simulink model "ROS"  (R2020b)
settings: Solver=FixedStepDiscrete  StartTime=start  StopTime=stop  FixedStep=T  MaxStep=0.01  RelTol=1e-3  EnableMultiTasking=on
model workspace (MAT data in the model file):
  SL_ROS_VariableLengthArrays_MaxSizes.CommonInfo.ArrayTruncateAction = 'EmitWarning'
  SL_ROS_VariableLengthArrays_MaxSizes.MsgTypeMap = containers.Map
  SL_ROS_VariableLengthArrays_MaxSizes.MsgTypeMap.serialization.keys = {'mav_msgs/Actuators'}
  SL_ROS_VariableLengthArrays_MaxSizes.MsgTypeMap.serialization.values{1}(1).PropertyName = 'Angles'
  SL_ROS_VariableLengthArrays_MaxSizes.MsgTypeMap.serialization.values{1}(1).DataType = 'double'
  SL_ROS_VariableLengthArrays_MaxSizes.MsgTypeMap.serialization.values{1}(1).MaxLength = 128
  SL_ROS_VariableLengthArrays_MaxSizes.MsgTypeMap.serialization.values{1}(2).PropertyName = 'AngularVelocities'
  SL_ROS_VariableLengthArrays_MaxSizes.MsgTypeMap.serialization.values{1}(2).DataType = 'double'
  SL_ROS_VariableLengthArrays_MaxSizes.MsgTypeMap.serialization.values{1}(2).MaxLength = 6
  SL_ROS_VariableLengthArrays_MaxSizes.MsgTypeMap.serialization.values{1}(3).PropertyName = 'Normalized'
  SL_ROS_VariableLengthArrays_MaxSizes.MsgTypeMap.serialization.values{1}(3).DataType = 'double'
  SL_ROS_VariableLengthArrays_MaxSizes.MsgTypeMap.serialization.values{1}(3).MaxLength = 128
  SL_ROS_VariableLengthArrays_MaxSizes.MsgTypeMap.serialization.uniformity = 0
  SL_ROS_VariableLengthArrays_MaxSizes.MsgTypeMap.serialization.keyType = 'char'
  SL_ROS_VariableLengthArrays_MaxSizes.MsgTypeMap.serialization.valueType = 'any'
values from neighbouring files (symbols this model uses):
  deltaOmegaNegBound = -1718    [ROS_Controller_Example.m]
  deltaOmegaPosBound = 1289    [ROS_Controller_Example.m]
  intAttPhi = intAttPhi_SIMULINK.signals.values(end)    [ROS_Controller_Example.m]
  intAttTheta = intAttTheta_SIMULINK.signals.values(end)    [ROS_Controller_Example.m]
  intPosXX = intPosXX_SIMULINK.signals.values(end)    [ROS_Controller_Example.m]
  intPosYY = intPosYY_SIMULINK.signals.values(end)    [ROS_Controller_Example.m]
  intRateRate = intRateRate_SIMULINK.signals.values(end)    [ROS_Controller_Example.m]
  intZZ = intZZ_SIMULINK.signals.values(end)    [ROS_Controller_Example.m]
  Kd_altitude = 373    [ROS_Controller_Example.m]
  Ki_altitude = 3.15    [ROS_Controller_Example.m]
  Ki_deltaPsi = 95.6839    [ROS_Controller_Example.m]
  Ki_pc = 0.0349    [ROS_Controller_Example.m]
  Ki_PhiC = -5.72958    [ROS_Controller_Example.m]
  Ki_qc = 0.0349    [ROS_Controller_Example.m]
  Ki_ThetaC = 5.72958    [ROS_Controller_Example.m]
  Kp_altitude = 70    [ROS_Controller_Example.m]
  Kp_deltaPhi = 1000    [ROS_Controller_Example.m]
  Kp_deltaPsi = 1000    [ROS_Controller_Example.m]
  Kp_deltaTheta = 1000    [ROS_Controller_Example.m]
  Kp_pc = 0.0611    [ROS_Controller_Example.m]
  Kp_PhiC = -3.594    [ROS_Controller_Example.m]
  Kp_qc = 0.0611    [ROS_Controller_Example.m]
  Kp_ThetaC = 3.594    [ROS_Controller_Example.m]
  Kp_YawPositionController = 0.0914    [ROS_Controller_Example.m]
  maxRotorsVelocity = 2618    [ROS_Controller_Example.m]
  motorAngularCoefficient = 0.2685    [ROS_Controller_Example.m]
  motorsIntercepts = 426.24    [ROS_Controller_Example.m]
  Omega_e = 6874    [ROS_Controller_Example.m]
  p_GAZEBO = msgS.Twist.Twist.Angular.X    [ROS_Controller_Example.m]
  phiCBound = pi/6    (= 0.523598775598)    [ROS_Controller_Example.m]
  pitch_MATLAB = EulerAngles(1,2)    [ROS_Controller_Example.m]
  psi_ref = 0    [ROS_Controller_Example.m]
  q_GAZEBO = msgS.Twist.Twist.Angular.Y    [ROS_Controller_Example.m]
  r_GAZEBO = msgS.Twist.Twist.Angular.Z    [ROS_Controller_Example.m]
  roll_MATLAB = EulerAngles(1,3)    [ROS_Controller_Example.m]
  T = 0.01    [ROS_Controller_Example.m]
  thetaCBound = pi/6    (= 0.523598775598)    [ROS_Controller_Example.m]
  u_GAZEBO = msgS.Twist.Twist.Linear.X    [ROS_Controller_Example.m]
  v_GAZEBO = msgS.Twist.Twist.Linear.Y    [ROS_Controller_Example.m]
  w_GAZEBO = msgS.Twist.Twist.Linear.Z    [ROS_Controller_Example.m]
  x_GAZEBO = msgS.Pose.Pose.Position.X    [ROS_Controller_Example.m]
  x_ref = 0    [ROS_Controller_Example.m]
  y_GAZEBO = msgS.Pose.Pose.Position.Y    [ROS_Controller_Example.m]
  y_ref = 0    [ROS_Controller_Example.m]
  yaw_MATLAB = EulerAngles(1,1)    [ROS_Controller_Example.m]
  yawRateBound = 3.4907    [ROS_Controller_Example.m]
  z_GAZEBO = msgS.Pose.Pose.Position.Z    [ROS_Controller_Example.m]
  z_ref = 1    [ROS_Controller_Example.m]
undefined symbols (not defined in the file or in its folder): DiscIntNeverNeededParam
settings Model: Creator=giuse  LastModifiedBy=FranciscoJose
settings DataIOCC: LimitDataPoints=on  SaveFormat=Array  ReturnWorkspaceOutputs=off
settings OptimizationCC: MaxStackSize=64
settings DebuggingCC: ParameterTunabilityLossMsg=error  ArithmeticOperatorsInVariantConditions=warning
settings HardwareCC: ProdBitPerPointer=32  ProdBitPerSizeT=32  ProdBitPerPtrDiffT=32  ProdLargestAtomicFloat=None  ProdIntDivRoundTo=Undefined  ProdEndianess=Unspecified  ProdWordSize=32  ProdHWDeviceType=Generic->Unspecified (assume 32-bit Generic)  UseEmbeddedCoderFeatures=off
settings ModelReferenceCC: PropagateSignalLabelsOutOfModel=off
settings SFSimCC: SimUseLocalCustomCode=off  CustomCodeUndefinedFunction=UseInterfaceOnly  SimTargetLang=C++
settings RTWCC: Description=Embedded Coder  SystemTargetFile=ert.tlc  HardwareBoard=Robot Operating System (ROS)  TLCOptions="-aInlineSetEventsForThisBaseRateFcn=TLC_FALSE -aSuppressMultiTaskScheduler=TLC_FALSE  -aRateBasedStepFcn=0"  TemplateMakefile=ert_default_tmf  GenerateReport=on  RTWUseLocalCustomCode=off  Toolchain=Catkin  LaunchReport=on  TargetLang=C++
settings CodeAppCC: ForceParamTrailComments=on  OperatorAnnotations=on  StateflowObjectComments=on  MATLABSourceComments=on
settings ERTTargetCC: MultiwordLength=2048  ERTCustomFileBanners=off  SupportContinuousTime=on  SupportNonInlinedSFcns=on  RemoveResetFunc=off  ModelStepFunctionPrototypeControlCompliant=off

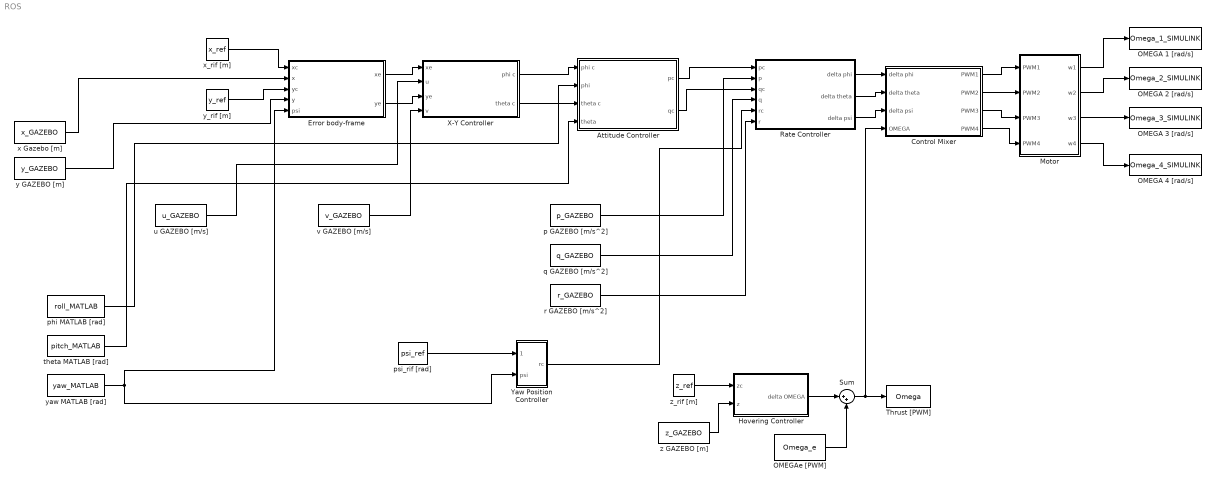
== system ROS ==
  Attitude Controller : Subsystem
  Control Mixer : Subsystem
  Error body-frame : Subsystem
  Hovering Controller : Subsystem
  Motor : Subsystem
  OMEGA 1 [rad/s] : ToWorkspace  VariableName=Omega_1_SIMULINK  SaveFormat=Structure With Time  SampleTime=-1
  OMEGA 2 [rad/s] : ToWorkspace  VariableName=Omega_2_SIMULINK  SaveFormat=Structure With Time  SampleTime=-1
  OMEGA 3 [rad/s] : ToWorkspace  VariableName=Omega_3_SIMULINK  SaveFormat=Structure With Time  SampleTime=-1
  OMEGA 4 [rad/s] : ToWorkspace  VariableName=Omega_4_SIMULINK  SaveFormat=Structure With Time  SampleTime=-1
  OMEGAe [PWM] : Constant  Value=Omega_e
  Rate Controller : Subsystem
  Sum : Sum  Inputs=|++
  Thrust [PWM] : ToWorkspace  VariableName=Omega  SaveFormat=Structure With Time  SampleTime=-1
  X-Y Controller : Subsystem
  Yaw Position Controller : Subsystem
  p GAZEBO [m/s^2] : Constant  Value=p_GAZEBO
  phi MATLAB [rad] : Constant  Value=roll_MATLAB
  psi_rif [rad] : Constant  Value=psi_ref
  q GAZEBO [m/s^2] : Constant  Value=q_GAZEBO
  r GAZEBO [m/s^2] : Constant  Value=r_GAZEBO
  theta MATLAB [rad] : Constant  Value=pitch_MATLAB
  u GAZEBO [m/s] : Constant  Value=u_GAZEBO
  v GAZEBO [m/s] : Constant  Value=v_GAZEBO
  x Gazebo [m] : Constant  Value=x_GAZEBO
  x_rif [m] : Constant  Value=x_ref
  y GAZEBO [m] : Constant  Value=y_GAZEBO
  y_rif [m] : Constant  Value=y_ref
  yaw MATLAB [rad] : Constant  Value=yaw_MATLAB
  z GAZEBO [m] : Constant  Value=z_GAZEBO
  z_rif [m] : Constant  Value=z_ref
  wires:
  Attitude Controller/2(qc) -> Rate Controller/3(qc)
  Control Mixer/1(PWM1) -> Motor/1(PWM1)
  Attitude Controller/1(pc) -> Rate Controller/1(pc)
  Control Mixer/2(PWM2) -> Motor/2(PWM2)
  Control Mixer/3(PWM3) -> Motor/3(PWM3)
  Control Mixer/4(PWM4) -> Motor/4(PWM4)
  Rate Controller/1(delta phi) -> Control Mixer/1(delta phi)
  Rate Controller/2(delta theta) -> Control Mixer/2(delta theta)
  Yaw Position Controller/1(rc) -> Rate Controller/5(rc)
  yaw MATLAB [rad]/1 -> Yaw Position Controller/2(psi), Error body-frame/5(psi)
  psi_rif [rad]/1 -> Yaw Position Controller/1(psi c)
  q GAZEBO [m/s^2]/1 -> Rate Controller/4(q)
  phi MATLAB [rad]/1 -> Attitude Controller/2(phi)
  z_rif [m]/1 -> Hovering Controller/1(zc)
  y_rif [m]/1 -> Error body-frame/3(yc)
  X-Y Controller/2(theta c) -> Attitude Controller/3(theta c)
  r GAZEBO [m/s^2]/1 -> Rate Controller/6(r)
  OMEGAe [PWM]/1 -> Sum/2
  X-Y Controller/1(phi c) -> Attitude Controller/1(phi c)
  Error body-frame/1(xe) -> X-Y Controller/1(xe)
  Hovering Controller/1(delta OMEGA) -> Sum/1
  Error body-frame/2(ye) -> X-Y Controller/3(ye)
  p GAZEBO [m/s^2]/1 -> Rate Controller/2(p)
  theta MATLAB [rad]/1 -> Attitude Controller/4(theta)
  x_rif [m]/1 -> Error body-frame/1(xc)
  Rate Controller/3(delta psi) -> Control Mixer/3(delta psi)
  Sum/1 -> Control Mixer/4(OMEGA), Thrust [PWM]/1
  x Gazebo [m]/1 -> Error body-frame/2(x)
  y GAZEBO [m]/1 -> Error body-frame/4(y)
  z GAZEBO [m]/1 -> Hovering Controller/2(z)
  u GAZEBO [m/s]/1 -> X-Y Controller/2(u)
  v GAZEBO [m/s]/1 -> X-Y Controller/4(v)
  Motor/3(w3) -> OMEGA 3 [rad/s]/1
  Motor/4(w4) -> OMEGA 4 [rad/s]/1
  Motor/2(w2) -> OMEGA 2 [rad/s]/1
  Motor/1(w1) -> OMEGA 1 [rad/s]/1

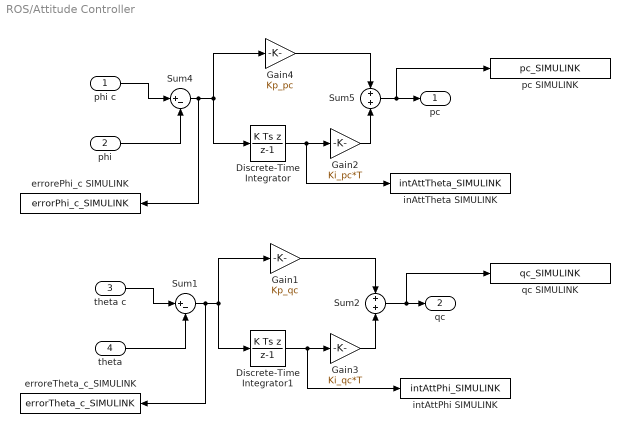
== system ROS/Attitude Controller ==
  phi c : Inport
  phi : Inport  Port=2
  theta c : Inport  Port=3
  theta : Inport  Port=4
  Discrete-Time Integrator : DiscreteIntegrator  IntegratorMethod=Integration: Backward Euler  gainval=1  InitialCondition=intAttPhi  SampleTime=-1  ICPrevOutput=DiscIntNeverNeededParam  ICPrevScaledInput=DiscIntNeverNeededParam
  Discrete-Time Integrator1 : DiscreteIntegrator  IntegratorMethod=Integration: Backward Euler  gainval=1  InitialCondition=intAttTheta  SampleTime=-1  ICPrevOutput=DiscIntNeverNeededParam  ICPrevScaledInput=DiscIntNeverNeededParam
  Gain1 : Gain  Gain=Kp_qc
  Gain2 : Gain  Gain=Ki_pc*T
  Gain3 : Gain  Gain=Ki_qc*T
  Gain4 : Gain  Gain=Kp_pc
  Sum1 : Sum  Inputs=|+-
  Sum2 : Sum
  Sum4 : Sum  Inputs=|+-
  Sum5 : Sum
  errorePhi_c SIMULINK : ToWorkspace  VariableName=errorPhi_c_SIMULINK  SaveFormat=Structure With Time  SampleTime=-1
  erroreTheta_c_SIMULINK : ToWorkspace  VariableName=errorTheta_c_SIMULINK  SaveFormat=Structure With Time  SampleTime=-1
  inAttTheta SIMULINK : ToWorkspace  VariableName=intAttTheta_SIMULINK  SaveFormat=Structure With Time  SampleTime=-1
  intAttPhi SIMULINK : ToWorkspace  VariableName=intAttPhi_SIMULINK  SaveFormat=Structure With Time  SampleTime=-1
  pc SIMULINK : ToWorkspace  VariableName=pc_SIMULINK  SaveFormat=Structure With Time  SampleTime=-1
  qc SIMULINK : ToWorkspace  VariableName=qc_SIMULINK  SaveFormat=Structure With Time  SampleTime=-1
  pc : Outport  VectorParamsAs1DForOutWhenUnconnected=off
  qc : Outport  Port=2  VectorParamsAs1DForOutWhenUnconnected=off
  wires:
  Gain4/1 -> Sum5/1
  Sum4/1 -> errorePhi_c SIMULINK/1, Discrete-Time Integrator/1, Gain4/1
  phi/1 -> Sum4/2
  Discrete-Time Integrator/1 -> inAttTheta SIMULINK/1, Gain2/1
  phi c/1 -> Sum4/1
  Sum5/1 -> pc SIMULINK/1, pc/1
  Gain1/1 -> Sum2/1
  Sum1/1 -> erroreTheta_c_SIMULINK/1, Discrete-Time Integrator1/1, Gain1/1
  theta/1 -> Sum1/2
  theta c/1 -> Sum1/1
  Sum2/1 -> qc SIMULINK/1, qc/1
  Gain2/1 -> Sum5/2
  Gain3/1 -> Sum2/2
  Discrete-Time Integrator1/1 -> intAttPhi SIMULINK/1, Gain3/1

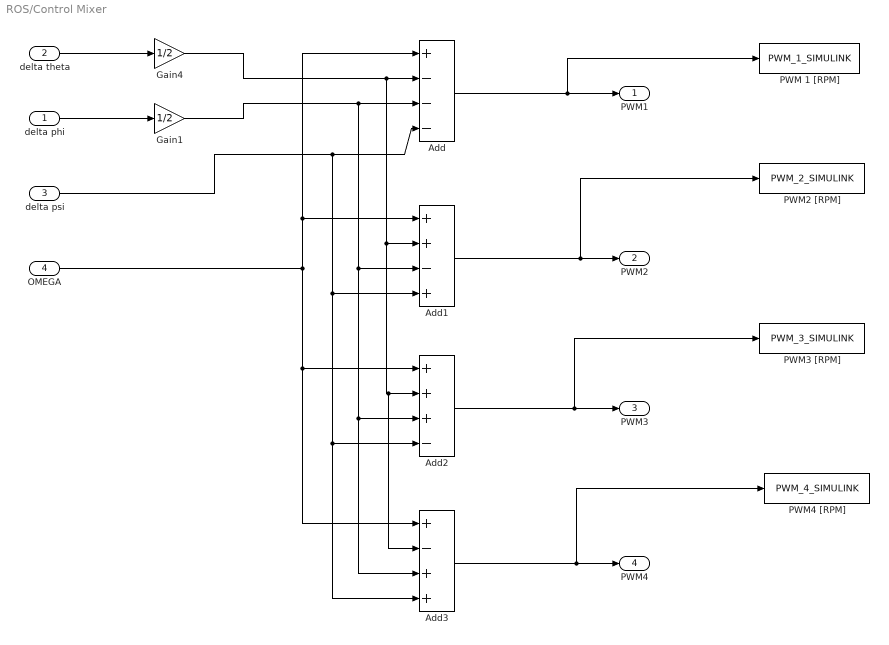
== system ROS/Control Mixer ==
  delta phi : Inport
  delta theta : Inport  Port=2
  delta psi : Inport  Port=3
  OMEGA : Inport  Port=4
  Add : Sum  Inputs=+---
  Add1 : Sum  Inputs=++-+
  Add2 : Sum  Inputs=+++-
  Add3 : Sum  Inputs=+-++
  Gain1 : Gain  Gain=1/2
  Gain4 : Gain  Gain=1/2
  PWM 1 [RPM] : ToWorkspace  VariableName=PWM_1_SIMULINK  SaveFormat=Structure With Time  SampleTime=-1
  PWM2 [RPM] : ToWorkspace  VariableName=PWM_2_SIMULINK  SaveFormat=Structure With Time  SampleTime=-1
  PWM3 [RPM] : ToWorkspace  VariableName=PWM_3_SIMULINK  SaveFormat=Structure With Time  SampleTime=-1
  PWM4 [RPM] : ToWorkspace  VariableName=PWM_4_SIMULINK  SaveFormat=Structure With Time  SampleTime=-1
  PWM1 : Outport  VectorParamsAs1DForOutWhenUnconnected=off
  PWM2 : Outport  Port=2  VectorParamsAs1DForOutWhenUnconnected=off
  PWM3 : Outport  Port=3  VectorParamsAs1DForOutWhenUnconnected=off
  PWM4 : Outport  Port=4  VectorParamsAs1DForOutWhenUnconnected=off
  wires:
  delta phi/1 -> Gain1/1
  OMEGA/1 -> Add1/1, Add/1, Add3/1, Add2/1
  Gain4/1 -> Add/2, Add1/2, Add3/2, Add2/2
  delta theta/1 -> Gain4/1
  delta psi/1 -> Add3/4, Add2/4, Add1/4, Add/4
  Gain1/1 -> Add/3, Add1/3, Add3/3, Add2/3
  Add/1 -> PWM 1 [RPM]/1, PWM1/1
  Add1/1 -> PWM2 [RPM]/1, PWM2/1
  Add2/1 -> PWM3 [RPM]/1, PWM3/1
  Add3/1 -> PWM4 [RPM]/1, PWM4/1

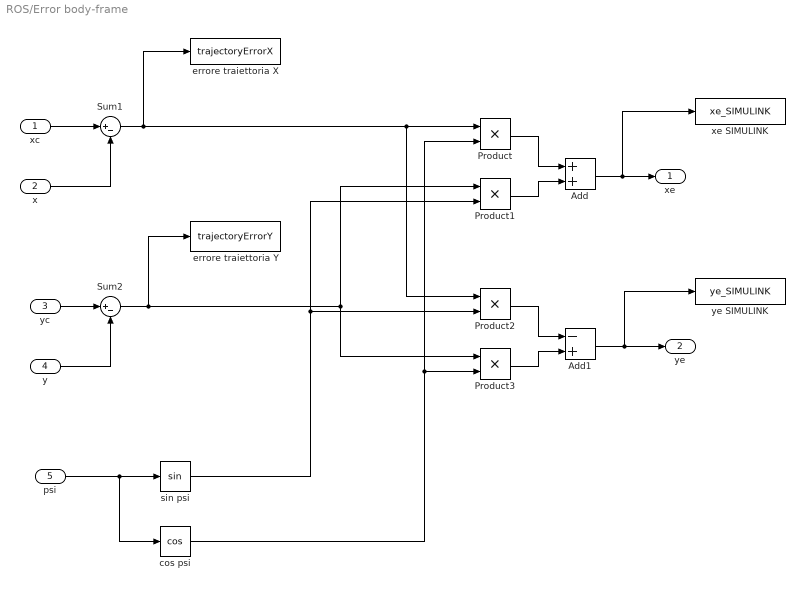
== system ROS/Error body-frame ==
  xc : Inport
  x : Inport  Port=2
  yc : Inport  Port=3
  y : Inport  Port=4
  psi : Inport  Port=5
  Add : Sum
  Add1 : Sum  Inputs=-+
  Product{,1..3} (4 alike) : Product
  Sum1 : Sum  Inputs=|+-
  Sum2 : Sum  Inputs=|+-
  cos psi : Trigonometry  Operator=cos
  errore traiettoria X : ToWorkspace  VariableName=trajectoryErrorX  SaveFormat=Structure With Time  SampleTime=-1
  errore traiettoria Y : ToWorkspace  VariableName=trajectoryErrorY  SaveFormat=Structure With Time  SampleTime=-1
  sin psi : Trigonometry
  xe SIMULINK : ToWorkspace  VariableName=xe_SIMULINK  SaveFormat=Structure With Time  SampleTime=-1
  ye SIMULINK : ToWorkspace  VariableName=ye_SIMULINK  SaveFormat=Structure With Time  SampleTime=-1
  xe : Outport  VectorParamsAs1DForOutWhenUnconnected=off
  ye : Outport  Port=2  VectorParamsAs1DForOutWhenUnconnected=off
  wires:
  x/1 -> Sum1/2
  xc/1 -> Sum1/1
  y/1 -> Sum2/2
  yc/1 -> Sum2/1
  psi/1 -> sin psi/1, cos psi/1
  Product1/1 -> Add/2
  Product/1 -> Add/1
  Product3/1 -> Add1/2
  Product2/1 -> Add1/1
  Sum1/1 -> errore traiettoria X/1, Product2/1, Product/1
  Sum2/1 -> Product3/1, Product1/1, errore traiettoria Y/1
  Add1/1 -> ye SIMULINK/1, ye/1
  Add/1 -> xe SIMULINK/1, xe/1
  cos psi/1 -> Product3/2, Product/2
  sin psi/1 -> Product2/2, Product1/2

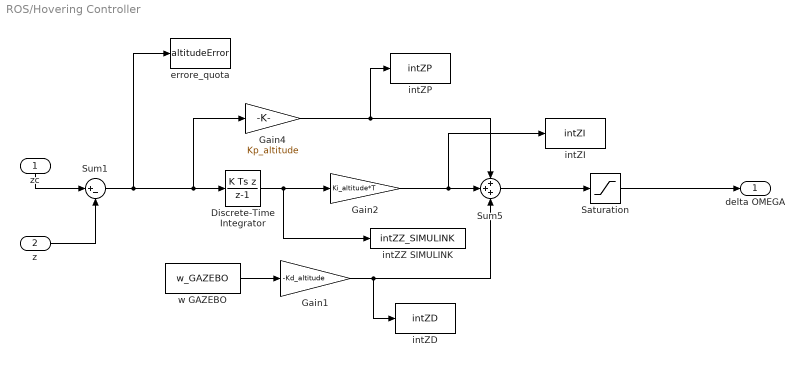
== system ROS/Hovering Controller ==
  zc : Inport
  z : Inport  Port=2
  Discrete-Time Integrator : DiscreteIntegrator  IntegratorMethod=Integration: Backward Euler  gainval=1  InitialCondition=intZZ  SampleTime=-1  ICPrevOutput=DiscIntNeverNeededParam  ICPrevScaledInput=DiscIntNeverNeededParam
  Gain1 : Gain  Gain=-Kd_altitude
  Gain2 : Gain  Gain=Ki_altitude*T
  Gain4 : Gain  Gain=Kp_altitude
  Saturation : Saturate  UpperLimit=deltaOmegaPosBound  LowerLimit=deltaOmegaNegBound
  Sum1 : Sum  Inputs=|+-
  Sum5 : Sum  Inputs=+++
  errore_quota : ToWorkspace  VariableName=altitudeError  SaveFormat=Structure With Time  SampleTime=-1
  intZD : ToWorkspace  VariableName=intZD  SaveFormat=Structure With Time  SampleTime=-1
  intZI : ToWorkspace  VariableName=intZI  SaveFormat=Structure With Time  SampleTime=-1
  intZP : ToWorkspace  VariableName=intZP  SaveFormat=Structure With Time  SampleTime=-1
  intZZ SIMULINK : ToWorkspace  VariableName=intZZ_SIMULINK  SaveFormat=Structure With Time  SampleTime=-1
  w GAZEBO : Constant  Value=w_GAZEBO
  delta OMEGA : Outport  VectorParamsAs1DForOutWhenUnconnected=off
  wires:
  Sum1/1 -> errore_quota/1, Discrete-Time Integrator/1, Gain4/1
  Gain4/1 -> intZP/1, Sum5/1
  z/1 -> Sum1/2
  zc/1 -> Sum1/1
  Gain1/1 -> intZD/1, Sum5/3
  Sum5/1 -> Saturation/1
  w GAZEBO/1 -> Gain1/1
  Saturation/1 -> delta OMEGA/1
  Discrete-Time Integrator/1 -> intZZ SIMULINK/1, Gain2/1
  Gain2/1 -> intZI/1, Sum5/2

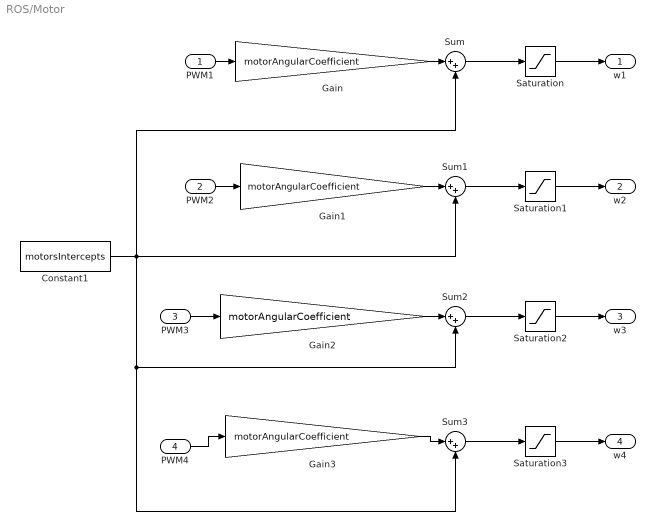
== system ROS/Motor ==
  PWM1 : Inport
  PWM2 : Inport  Port=2
  PWM3 : Inport  Port=3
  PWM4 : Inport  Port=4
  Constant1 : Constant  Value=motorsIntercepts
  Gain{,1..3} (4 alike) : Gain  Gain=motorAngularCoefficient
  Saturation{,1..3} (4 alike) : Saturate  UpperLimit=maxRotorsVelocity  LowerLimit=0
  Sum{,1..3} (4 alike) : Sum  Inputs=|++
  w1 : Outport  VectorParamsAs1DForOutWhenUnconnected=off
  w2 : Outport  Port=2  VectorParamsAs1DForOutWhenUnconnected=off
  w3 : Outport  Port=3  VectorParamsAs1DForOutWhenUnconnected=off
  w4 : Outport  Port=4  VectorParamsAs1DForOutWhenUnconnected=off
  wires:
  Gain/1 -> Sum/1
  PWM1/1 -> Gain/1
  Gain1/1 -> Sum1/1
  PWM2/1 -> Gain1/1
  Gain2/1 -> Sum2/1
  PWM3/1 -> Gain2/1
  Gain3/1 -> Sum3/1
  PWM4/1 -> Gain3/1
  Constant1/1 -> Sum1/2, Sum2/2, Sum3/2, Sum/2
  Sum/1 -> Saturation/1
  Sum1/1 -> Saturation1/1
  Sum2/1 -> Saturation2/1
  Sum3/1 -> Saturation3/1
  Saturation/1 -> w1/1
  Saturation1/1 -> w2/1
  Saturation2/1 -> w3/1
  Saturation3/1 -> w4/1

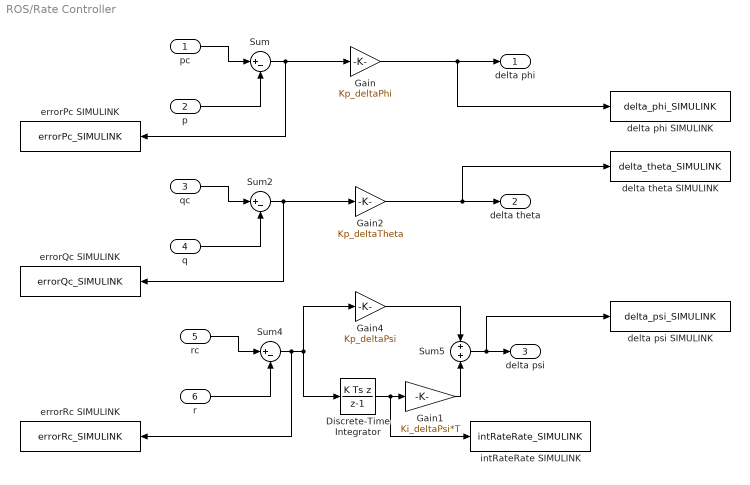
== system ROS/Rate Controller ==
  pc : Inport
  p : Inport  Port=2
  qc : Inport  Port=3
  q : Inport  Port=4
  rc : Inport  Port=5
  r : Inport  Port=6
  Discrete-Time Integrator : DiscreteIntegrator  IntegratorMethod=Integration: Backward Euler  gainval=1  InitialCondition=intRateRate  SampleTime=-1  ICPrevOutput=DiscIntNeverNeededParam  ICPrevScaledInput=DiscIntNeverNeededParam
  Gain : Gain  Gain=Kp_deltaPhi
  Gain1 : Gain  Gain=Ki_deltaPsi*T
  Gain2 : Gain  Gain=Kp_deltaTheta
  Gain4 : Gain  Gain=Kp_deltaPsi
  Sum : Sum  Inputs=|+-
  Sum2 : Sum  Inputs=|+-
  Sum4 : Sum  Inputs=|+-
  Sum5 : Sum
  delta phi SIMULINK : ToWorkspace  VariableName=delta_phi_SIMULINK  SaveFormat=Structure With Time  SampleTime=-1
  delta psi SIMULINK : ToWorkspace  VariableName=delta_psi_SIMULINK  SaveFormat=Structure With Time  SampleTime=-1
  delta theta SIMULINK : ToWorkspace  VariableName=delta_theta_SIMULINK  SaveFormat=Structure With Time  SampleTime=-1
  errorPc SIMULINK : ToWorkspace  VariableName=errorPc_SIMULINK  SaveFormat=Structure With Time  SampleTime=-1
  errorQc SIMULINK : ToWorkspace  VariableName=errorQc_SIMULINK  SaveFormat=Structure With Time  SampleTime=-1
  errorRc SIMULINK : ToWorkspace  VariableName=errorRc_SIMULINK  SaveFormat=Structure With Time  SampleTime=-1
  intRateRate SIMULINK : ToWorkspace  VariableName=intRateRate_SIMULINK  SaveFormat=Structure With Time  SampleTime=-1
  delta phi : Outport  VectorParamsAs1DForOutWhenUnconnected=off
  delta theta : Outport  Port=2  VectorParamsAs1DForOutWhenUnconnected=off
  delta psi : Outport  Port=3  VectorParamsAs1DForOutWhenUnconnected=off
  wires:
  Sum/1 -> errorPc SIMULINK/1, Gain/1
  p/1 -> Sum/2
  pc/1 -> Sum/1
  Gain/1 -> delta phi SIMULINK/1, delta phi/1
  Sum2/1 -> errorQc SIMULINK/1, Gain2/1
  q/1 -> Sum2/2
  qc/1 -> Sum2/1
  Gain2/1 -> delta theta SIMULINK/1, delta theta/1
  Gain4/1 -> Sum5/1
  Sum4/1 -> errorRc SIMULINK/1, Discrete-Time Integrator/1, Gain4/1
  r/1 -> Sum4/2
  Discrete-Time Integrator/1 -> intRateRate SIMULINK/1, Gain1/1
  rc/1 -> Sum4/1
  Sum5/1 -> delta psi SIMULINK/1, delta psi/1
  Gain1/1 -> Sum5/2

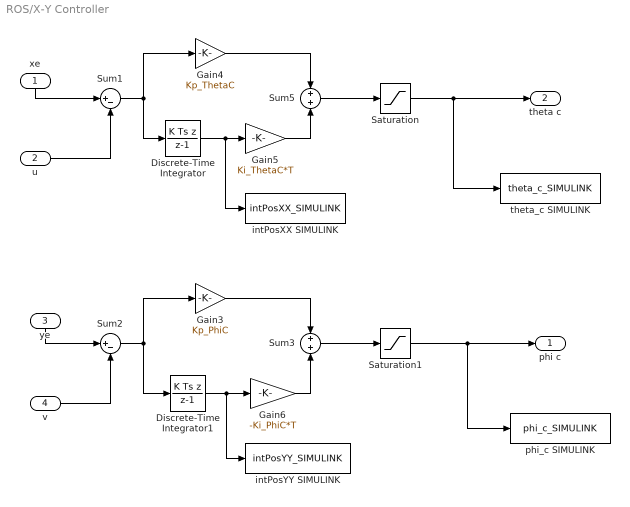
== system ROS/X-Y Controller ==
  xe : Inport
  u : Inport  Port=2
  ye : Inport  Port=3
  v : Inport  Port=4
  Discrete-Time Integrator : DiscreteIntegrator  IntegratorMethod=Integration: Backward Euler  gainval=1  InitialCondition=intPosXX  SampleTime=-1  ICPrevOutput=DiscIntNeverNeededParam  ICPrevScaledInput=DiscIntNeverNeededParam
  Discrete-Time Integrator1 : DiscreteIntegrator  IntegratorMethod=Integration: Backward Euler  gainval=1  InitialCondition=intPosYY  SampleTime=-1  ICPrevOutput=DiscIntNeverNeededParam  ICPrevScaledInput=DiscIntNeverNeededParam
  Gain3 : Gain  Gain=Kp_PhiC
  Gain4 : Gain  Gain=Kp_ThetaC
  Gain5 : Gain  Gain=Ki_ThetaC*T
  Gain6 : Gain  Gain=-Ki_PhiC*T
  Saturation : Saturate  UpperLimit=thetaCBound  LowerLimit=-thetaCBound
  Saturation1 : Saturate  UpperLimit=phiCBound  LowerLimit=-phiCBound
  Sum1 : Sum  Inputs=|+-
  Sum2 : Sum  Inputs=|+-
  Sum3 : Sum
  Sum5 : Sum
  intPosXX SIMULINK : ToWorkspace  VariableName=intPosXX_SIMULINK  SaveFormat=Structure With Time  SampleTime=-1
  intPosYY SIMULINK : ToWorkspace  VariableName=intPosYY_SIMULINK  SaveFormat=Structure With Time  SampleTime=-1
  phi_c SIMULINK : ToWorkspace  VariableName=phi_c_SIMULINK  SaveFormat=Structure With Time  SampleTime=-1
  theta_c SIMULINK : ToWorkspace  VariableName=theta_c_SIMULINK  SaveFormat=Structure With Time  SampleTime=-1
  phi c : Outport  VectorParamsAs1DForOutWhenUnconnected=off
  theta c : Outport  Port=2  VectorParamsAs1DForOutWhenUnconnected=off
  wires:
  Gain4/1 -> Sum5/1
  Discrete-Time Integrator/1 -> intPosXX SIMULINK/1, Gain5/1
  Sum5/1 -> Saturation/1
  xe/1 -> Sum1/1
  Sum1/1 -> Discrete-Time Integrator/1, Gain4/1
  Gain5/1 -> Sum5/2
  Gain6/1 -> Sum3/2
  Sum2/1 -> Discrete-Time Integrator1/1, Gain3/1
  Sum3/1 -> Saturation1/1
  Gain3/1 -> Sum3/1
  Discrete-Time Integrator1/1 -> intPosYY SIMULINK/1, Gain6/1
  ye/1 -> Sum2/1
  Saturation/1 -> theta_c SIMULINK/1, theta c/1
  Saturation1/1 -> phi_c SIMULINK/1, phi c/1
  u/1 -> Sum1/2
  v/1 -> Sum2/2

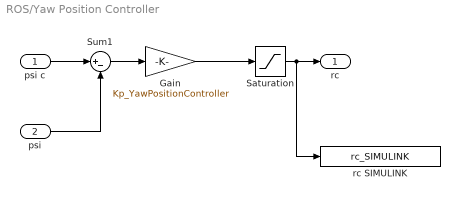
== system ROS/Yaw Position Controller ==
  psi c : Inport
  psi : Inport  Port=2
  Gain : Gain  Gain=Kp_YawPositionController
  Saturation : Saturate  UpperLimit=yawRateBound  LowerLimit=-yawRateBound
  Sum1 : Sum  Inputs=|+-
  rc SIMULINK : ToWorkspace  VariableName=rc_SIMULINK  SaveFormat=Structure With Time  SampleTime=-1
  rc : Outport  VectorParamsAs1DForOutWhenUnconnected=off
  wires:
  psi c/1 -> Sum1/1
  Sum1/1 -> Gain/1
  Gain/1 -> Saturation/1
  psi/1 -> Sum1/2
  Saturation/1 -> rc SIMULINK/1, rc/1
